simulink model "SEA_system"  (R2023b)
settings: Solver=VariableStepAuto  StartTime=0.0  StopTime=30  RelTol=1e-3
values from neighbouring files (symbols this model uses):
  c1 = 0.05    [SEA_system.m]
  c2 = 0.05    [SEA_system.m]
  Fx = 0    [SEA_system.m]
  Fy = 0    [SEA_system.m]
  J1 = m1*L1^2/12 + m1*CoM1^2    (= 0.00579610927083)    [SEA_system.m]
  J2 = m2*L2^2/12 + m2*CoM2^2 + (mEE*(L2-CoM2)^2)    (= 0.00129963166667)    [SEA_system.m]
  k1 = 5.9*10^3    (= 5900)    [SEA_system.m]
  k2 = 5.9*10^3    (= 5900)    [SEA_system.m]
  L1 = 0.20075    [SEA_system.m]
  L2 = 0.149    [SEA_system.m]
libraries: simulink_extras x2
settings Model: Creator=Master  LastModifiedBy=Master

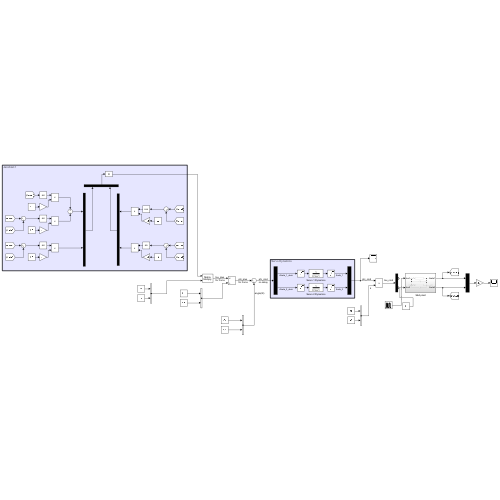
[thumbnail: Simulink's stored preview of the top-level diagram]
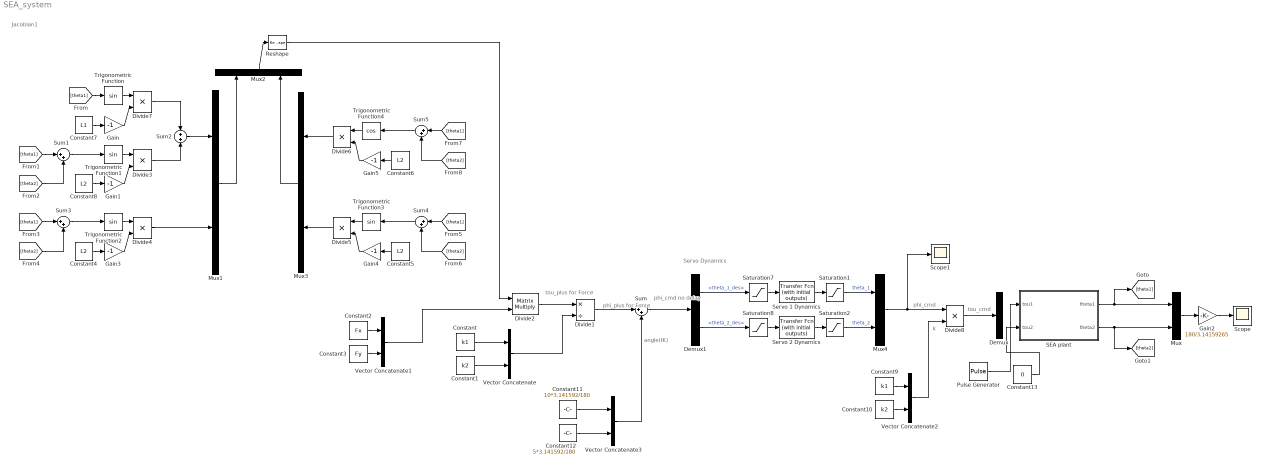
== system SEA_system ==
  note: tou_plus
      | for Force
  note: angle(IK)
  note: Servo Dynamics
  note: Jacobian1
  note: tou_cmd
  note: k
  note: phi_cmd
  note: phi_cmd
      | no delay
  note: phi_plus
      | for Force
  Constant : Constant  Value=k1
  Constant1 : Constant  Value=k2
  Constant10 : Constant  Value=k2
  Constant11 : Constant  Value=10*3.141592/180
  Constant12 : Constant  Value=5*3.141592/180
  Constant13 : Constant  Value=0
  Constant2 : Constant  Value=Fx
  Constant3 : Constant  Value=Fy
  Constant{4..6,8} (4 alike) : Constant  Value=L2
  Constant7 : Constant  Value=L1
  Constant9 : Constant  Value=k1
  Demux : Demux  Outputs=2
  Demux1 : Demux  Outputs=2
  Divide1 : Product  Inputs=*/
  Divide2 : Product  Inputs=**  Multiplication=Matrix(*)
  Divide{3..8} (6 alike) : Product  Inputs=**
  Gain{,1,3..5} (5 alike) : Gain  Gain=-1
  Gain2 : Gain  Gain=180/3.14159265
  Mux{,1..4} (5 alike) : Mux  Inputs=2
  Pulse Generator : DiscretePulseGenerator  PulseType=Time based  Amplitude=10  Period=30  PulseWidth=10  PhaseDelay=10
  Reshape : Reshape  OutputDimensionality=Customize  OutputDimensions=[2,2]
  SEA plant : Subsystem
  Saturation{1..2,7..8} (4 alike) : Saturate  UpperLimit=0.3  LowerLimit=-0.3
  Scope : Scope
  Scope1 : Scope
  Servo 1 Dynamics : simulink_extras/Additional Linear/Transfer Fcn (with initial outputs)  N=[1]  D="[1/10  1]"  Y0=0  U0=0
  Servo 2 Dynamics : simulink_extras/Additional Linear/Transfer Fcn (with initial outputs)  N=[1]  D="[1/10  1]"  Y0=0  U0=0
  Sum{,1,3..5} (5 alike) : Sum  Inputs=|++
  Sum2 : Sum  Inputs=+|+
  Trigonometric Function{,1..3} (4 alike) : Trigonometry
  Trigonometric Function4 : Trigonometry  Operator=cos
  Vector Concatenate{,1..3} (4 alike) : Concatenate
  wires:
  Gain2/1 -> Scope/1
  Mux/1 -> Gain2/1
  SEA plant/1(theta1) -> [theta1], Mux/1
  SEA plant/2(theta2) -> [theta2], Mux/2
  Divide1/1 -> Sum/1
  Constant/1 -> Vector Concatenate/1
  Constant1/1 -> Vector Concatenate/2
  Divide2/1 -> Divide1/1
  Constant3/1 -> Vector Concatenate1/2
  Constant2/1 -> Vector Concatenate1/1
  Vector Concatenate1/1 -> Divide2/2
  Vector Concatenate/1 -> Divide1/2
  Reshape/1 -> Divide2/1
  [theta2] -> Sum5/2
  [theta1] -> Sum4/1
  Gain1/1 -> Divide3/2
  [theta1] -> Trigonometric Function/1
  Gain3/1 -> Divide4/2
  Trigonometric Function4/1 -> Divide6/1
  Constant8/1 -> Gain1/1
  [theta2] -> Sum1/2
  Constant7/1 -> Gain/1
  Trigonometric Function1/1 -> Divide3/1
  Constant6/1 -> Gain5/1
  Trigonometric Function3/1 -> Divide5/1
  Sum5/1 -> Trigonometric Function4/1
  Gain/1 -> Divide7/2
  Divide6/1 -> Mux3/1
  Sum3/1 -> Trigonometric Function2/1
  Constant5/1 -> Gain4/1
  [theta2] -> Sum4/2
  Mux1/1 -> Mux2/1
  Gain5/1 -> Divide6/2
  Sum4/1 -> Trigonometric Function3/1
  [theta1] -> Sum5/1
  Sum1/1 -> Trigonometric Function1/1
  Constant4/1 -> Gain3/1
  Sum2/1 -> Mux1/1
  Divide7/1 -> Sum2/1
  Trigonometric Function/1 -> Divide7/1
  [theta1] -> Sum1/1
  Divide3/1 -> Sum2/2
  Mux3/1 -> Mux2/2
  [theta1] -> Sum3/1
  Trigonometric Function2/1 -> Divide4/1
  [theta2] -> Sum3/2
  Divide4/1 -> Mux1/2
  Divide5/1 -> Mux3/2
  Gain4/1 -> Divide5/2
  Mux2/1 -> Reshape/1
  Vector Concatenate2/1 -> Divide8/2
  Constant10/1 -> Vector Concatenate2/2
  Constant9/1 -> Vector Concatenate2/1
  Sum/1 -> Demux1/1
  Servo 1 Dynamics/1 -> Saturation1/1
  Servo 2 Dynamics/1 -> Saturation2/1
  Saturation7/1 -> Servo 1 Dynamics/1
  Demux1/2 -> Saturation8/1  "<theta_2_des>"
  Demux1/1 -> Saturation7/1  "<theta_1_des>"
  Saturation8/1 -> Servo 2 Dynamics/1
  Saturation1/1 -> Mux4/1  "theta_1"
  Saturation2/1 -> Mux4/2  "theta_2"
  Mux4/1 -> Scope1/1, Divide8/1
  Vector Concatenate3/1 -> Sum/2
  Constant12/1 -> Vector Concatenate3/2
  Constant11/1 -> Vector Concatenate3/1
  Divide8/1 -> Demux/1
  Pulse Generator/1 -> SEA plant/1(tou1)
  Constant13/1 -> SEA plant/2(tou2)

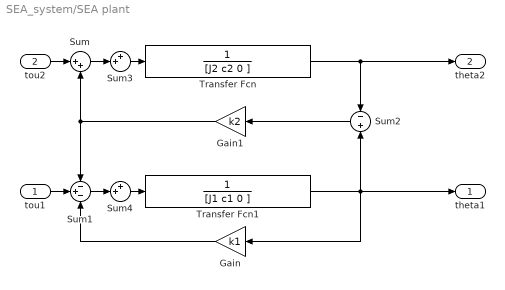
== system SEA_system/SEA plant ==
  tou1 : Inport
  tou2 : Inport  Port=2
  Gain : Gain  Gain=k1
  Gain1 : Gain  Gain=k2
  Sum : Sum  Inputs=|++
  Sum1 : Sum  Inputs=-+-
  Sum2 : Sum  Inputs=-|+
  Sum3 : Sum  Inputs=++|
  Sum4 : Sum  Inputs=++|
  Transfer Fcn : TransferFcn  Denominator=[J2 c2 0 ]
  Transfer Fcn1 : TransferFcn  Denominator=[J1 c1 0 ]
  theta1 : Outport
  theta2 : Outport  Port=2
  wires:
  Gain1/1 -> Sum1/1, Sum/2
  Transfer Fcn1/1 -> Sum2/2, theta1/1, Gain/1
  Sum2/1 -> Gain1/1
  tou1/1 -> Sum1/2
  Transfer Fcn/1 -> theta2/1, Sum2/1
  Gain/1 -> Sum1/3
  tou2/1 -> Sum/1
  Sum/1 -> Sum3/2
  Sum3/1 -> Transfer Fcn/1
  Sum1/1 -> Sum4/2
  Sum4/1 -> Transfer Fcn1/1
